simulink model "hp_v5"  (R2024a)
settings: Solver=VariableStepAuto  StartTime=0.0  StopTime=tf  MaxStep=1e-4  RelTol=1e-3  AbsTol=1e-4
values from neighbouring files (symbols this model uses):
  coupler = hexapod.coupler    [calcMotorAngles.m]    (also in calcMotorAngles2.m; calcMotorAngles3.m; calcQ.m; calcQ2_bak.m)
  D = 2 * zeta * w_n * J_e    [controller_parameters.m]    (also in main.m; main_feedforward.m)
  excenter = hexapod.excenter    [calcMotorAngles.m]    (also in calcMotorAngles2.m; calcMotorAngles3.m; calcQ.m; calcQ2_bak.m)
  linear_spring_length = 1    [main.m]    (also in main_feedforward.m = 10)
  linear_spring_offset = ((((platform_mass + 6 * coupler_mass+ 6 * excenter_mass/2) * g)) / linear_spring_constant)    [main.m]    (also in main_feedforward.m = ((platform_mass + 6*coupler_mass+ 6 * excenter_mass/2) * g) )
  motorData = [time0, -motorAngles(:,1), -motorAngles(:,2),                -motorAngles(:,3), -motorAngles(:,4),                -motorAngles(:,5), -motorAngles(:,6)]    [calcSpringParam.m]    (also in calc_spring_param.m; generateMotorDataFromFile.m = [time0, -motorAngles(:,1), -motorAngles(:,2),               ; generateMotorDataFromTrajFile.m = [time0, -motorAngles(:,1), -motorAngles(:,2),               ; generateMotorDataJog.m = [time0, -motorAngles(:,1), -motorAngles(:,2),               )
  N = size(M, 1)    [generateMotorDataFromFile.m]    (also in generateMotorDataFromTrajFile.m; main.m = 36; main_feedforward.m = 36; rw.m = size(data, 1))
  P = w_n^2 * J_e - K_e    [controller_parameters.m]    (also in main.m; main_feedforward.m)
  q = q_rots    [q_test.m]
  radius = 0.01    [main.m]    (also in main_feedforward.m)
  w_f = w_n *10    (= 942.477796077)    [controller_parameters.m]    (also in main.m = 837.758040957; main_feedforward.m = 837.758040957)
  Y = fft(motorAnglesmask(:, col))    [calc_spring_param.m]
undefined symbols (not defined in the file or in its folder): X, y_zero, Z
libraries: nesl_utility x54, sm_lib x48
(part 2 of 2)

== system hp_v5/Lookup tables ==
  1-D Lookup Table : Lookup_n-D  NumberOfTableDimensions=1  BreakpointsForDimension1=motorData(:,1)  Table=motorData(:,2)  InterpMethod=Cubic spline  InternalRulePriority=Speed  RndMeth=Simplest
  1-D Lookup Table1 : Lookup_n-D  NumberOfTableDimensions=1  BreakpointsForDimension1=motorData(:,1)  Table=motorData(:,3)  InterpMethod=Cubic spline  InternalRulePriority=Speed  RndMeth=Simplest
  1-D Lookup Table2 : Lookup_n-D  NumberOfTableDimensions=1  BreakpointsForDimension1=motorData(:,1)  Table=motorData(:,4)  InterpMethod=Cubic spline  InternalRulePriority=Speed  RndMeth=Simplest
  1-D Lookup Table3 : Lookup_n-D  NumberOfTableDimensions=1  BreakpointsForDimension1=motorData(:,1)  Table=motorData(:,5)  InterpMethod=Cubic spline  InternalRulePriority=Speed  RndMeth=Simplest
  1-D Lookup Table4 : Lookup_n-D  NumberOfTableDimensions=1  BreakpointsForDimension1=motorData(:,1)  Table=motorData(:,6)  InterpMethod=Cubic spline  InternalRulePriority=Speed  RndMeth=Simplest
  1-D Lookup Table5 : Lookup_n-D  NumberOfTableDimensions=1  BreakpointsForDimension1=motorData(:,1)  Table=motorData(:,7)  InterpMethod=Cubic spline  InternalRulePriority=Speed  RndMeth=Simplest
  Clock : Clock
  Mux1 : Mux  Inputs=6
  Angles : Outport
  wires:
  Mux1/1 -> Angles/1
  1-D Lookup Table5/1 -> Mux1/6  "lookup"
  1-D Lookup Table3/1 -> Mux1/4  "lookup"
  1-D Lookup Table1/1 -> Mux1/2  "lookup"
  Clock/1 -> 1-D Lookup Table/1, 1-D Lookup Table1/1, 1-D Lookup Table2/1, 1-D Lookup Table5/1, 1-D Lookup Table4/1, 1-D Lookup Table3/1
  1-D Lookup Table4/1 -> Mux1/5  "lookup"
  1-D Lookup Table2/1 -> Mux1/3  "lookup"
  1-D Lookup Table/1 -> Mux1/1  "lookup"

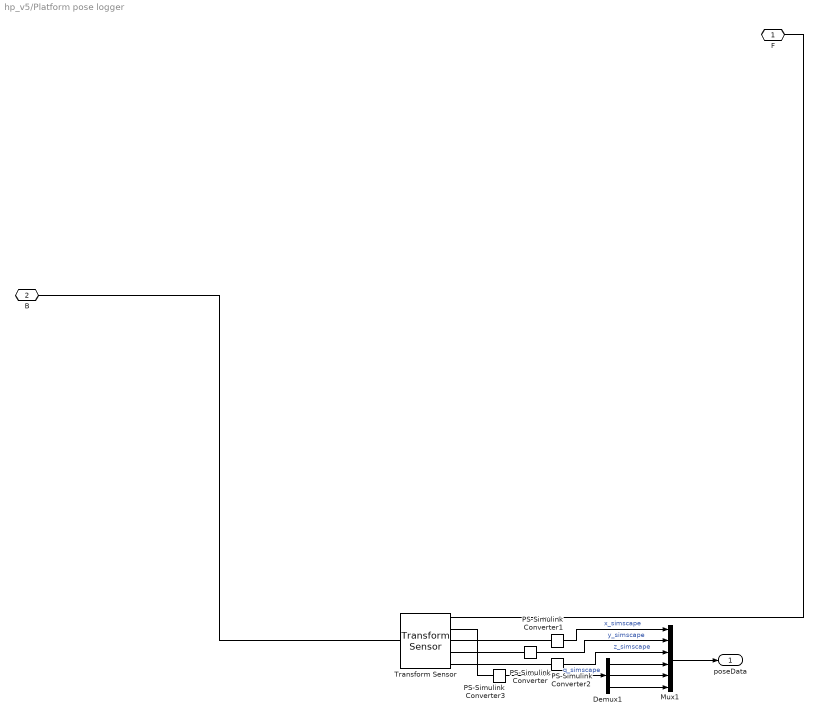
== system hp_v5/Platform pose logger ==
  Demux1 : Demux  Outputs=3
  Mux1 : Mux  Inputs=6
  PS-Simulink Converter{,1..3} (4 alike) : nesl_utility/PS-Simulink Converter  PhysicalDomain=network_engine_domain  SubClassName=ps_output  LeftPortType=input  RightPortType=output  PseudoPeriodic=off  Frequencies=[]  VectorFormat=inherit  Unit=inherit  AffineConversion=off
  Transform Sensor : sm_lib/Frames and Transforms/Transform Sensor  MeasurementFrame=World  RotationSequence=XYZ  SenseAngle=off  SenseAxis=off  SenseQ=off  SenseR=off  SenseRotationSequence=on  SenseOmegaX=off  SenseOmegaY=off  SenseOmegaZ=off  SenseOmega=off  SenseQDot=off  SenseRDot=off  SenseRotationSequenceDot=off  SenseAlphaX=off  SenseAlphaY=off  SenseAlphaZ=off  SenseAlpha=off  SenseQDDot=off  SenseRDDot=off  SenseX=on  SenseY=on  SenseZ=on  SenseXYZ=off  SenseRad=off  SenseAzim=off  SenseDist=off  SenseInc=off  SenseXDot=off  SenseYDot=off  SenseZDot=off  SenseXYZDot=off  SenseRadDot=off  SenseAzimDot=off  SenseDistDot=off  SenseIncDot=off  SenseXDDot=off  SenseYDDot=off  SenseZDDot=off  SenseXYZDDot=off  SenseRadDDot=off  SenseAzimDDot=off  SenseDistDDot=off  SenseIncDDot=off
  F : PMIOPort  Side=Right
  B : PMIOPort  Port=2  Side=Left
  poseData : Outport
  wires:
  Demux1/1 -> Mux1/4
  Demux1/2 -> Mux1/5
  Demux1/3 -> Mux1/6
  PS-Simulink Converter/1 -> Mux1/2  "y_simscape"
  PS-Simulink Converter2/1 -> Mux1/3  "z_simscape"
  PS-Simulink Converter1/1 -> Mux1/1  "x_simscape"
  PS-Simulink Converter3/1 -> Demux1/1  "q_simscape"
  Mux1/1 -> poseData/1
  connections:
  PS-Simulink Converter2/LConn1 -- Transform Sensor/RConn5
  PS-Simulink Converter/LConn1 -- Transform Sensor/RConn4
  PS-Simulink Converter1/LConn1 -- Transform Sensor/RConn3
  PS-Simulink Converter3/LConn1 -- Transform Sensor/RConn2
  Transform Sensor/LConn1 -- B/RConn1
  F/RConn1 -- Transform Sensor/RConn1

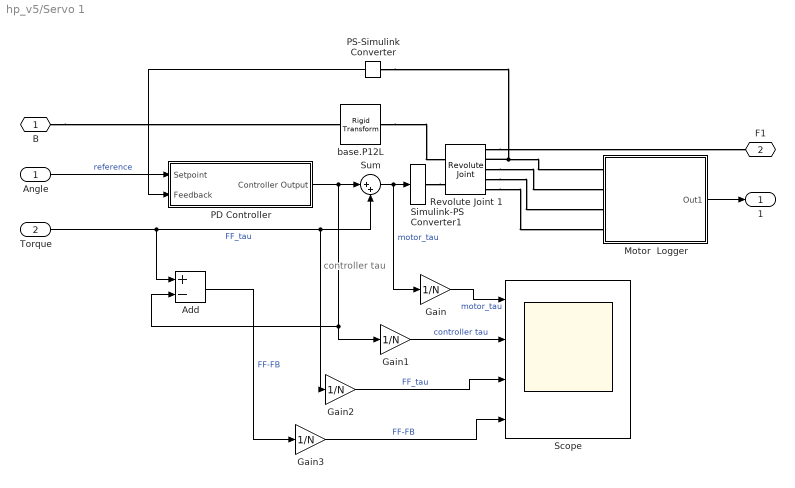
== system hp_v5/Servo 1 ==
  note: controller tau
  Angle : Inport
  Torque : Inport  Port=2
  Add : Sum  Inputs=+-
  Gain{,1..3} (4 alike) : Gain  Gain=1/N
  Motor  Logger : Subsystem
  PD Controller : Subsystem
  PS-Simulink Converter : nesl_utility/PS-Simulink Converter  PhysicalDomain=network_engine_domain  SubClassName=ps_output  LeftPortType=input  RightPortType=output  PseudoPeriodic=off  Frequencies=[]  VectorFormat=inherit  Unit=inherit  AffineConversion=off
  Revolute Joint 1 : sm_lib/Joints/Revolute Joint  JointMode=Normal  CompositeWrenchDir=FollowerOnBase  CompositeWrenchFrame=BaseFrame  SenseConstraintForce=off  SenseConstraintTorque=off  SenseTotalForce=off  SenseTotalTorque=off  PositionTargetSpecify=off  PositionTargetPriority=High  PositionTargetValue=0  PositionTargetValueUnits=deg  VelocityTargetSpecify=off  VelocityTargetPriority=High  VelocityTargetValue=0  VelocityTargetValueUnits=deg/s  EquilibriumPosition=0  EquilibriumPositionUnits=rad  SpringStiffness=0  SpringStiffnessUnits=N*m/rad  DampingCoefficient=0  DampingCoefficientUnits=N*m*s/rad  LowerLimitSpecify=off  LowerLimitBound=-90  LowerLimitBoundUnits=deg  LowerLimitStiffness=1e4  LowerLimitStiffnessUnits=N*m/deg  LowerLimitDamping=10  LowerLimitDampingUnits=N*m/(deg/s)  LowerLimitTransitionRegionWidth=0.1  LowerLimitTransitionRegionWidthUnits=deg  UpperLimitSpecify=off  UpperLimitBound=90  UpperLimitBoundUnits=deg  UpperLimitStiffness=1e4  UpperLimitStiffnessUnits=N*m/deg  UpperLimitDamping=10  UpperLimitDampingUnits=N*m/(deg/s)  UpperLimitTransitionRegionWidth=0.1  UpperLimitTransitionRegionWidthUnits=deg  TorqueActuationMode=InputTorque  MotionActuationMode=ComputedMotion  SensePosition=on  SenseVelocity=on  SenseAcceleration=on  SenseTorqueForce=on  SenseLowerLimitTorqueForce=off  SenseUpperLimitTorqueForce=off
  Scope : Scope  NumInputPorts=4
  Simulink-PS Converter1 : nesl_utility/Simulink-PS Converter  PhysicalDomain=network_engine_domain  SubClassName=ps_input  LeftPortType=input  RightPortType=output  PseudoPeriodic=off  Frequencies=[]  NoiseDistribution=none  NoiseParameters=[]  Unit=1  AffineConversion=off  FilteringAndDerivatives=filter  SimscapeFilterOrder=2  InputFilterTimeConstant=0.001  UdotUserProvided=1
  Sum : Sum  Inputs=|++
  base.P12L : sm_lib/Frames and Transforms/Rigid Transform  RotationMethod=StandardAxis  FollAlignAxisA=+X  BaseAlignAxisA=+Y  FollAlignAxisB=+Y  BaseAlignAxisB=+Z  RotationStandardAxis=+Y  RotationAngle=-120  RotationAngleUnits=deg  RotationArbitraryAxis=[0 0 1]  RotationSequenceAxes=FollowerAxes  RotationSequence=XYX  RotationSequenceAngles=[0 0 0]  RotationSequenceAnglesUnits=deg  RotationMatrix=[1 0 0;0 1 0;0 0 1]  Quaternion=[1 0 0 0]  TranslationMethod=Cartesian  TranslationCartesianOffset=base.P12L  TranslationCartesianOffsetUnits=m  TranslationStandardAxis=+Z  TranslationStandardOffset=0  TranslationStandardOffsetUnits=m  TranslationROffset=0  TranslationROffsetUnits=m  TranslationThetaOffset=0  TranslationThetaOffsetUnits=deg  TranslationZOffset=0  TranslationZOffsetUnits=m
  B : PMIOPort  Side=Left
  F1 : PMIOPort  Port=2  Side=Right
  1 : Outport
  wires:
  PS-Simulink Converter/1 -> PD Controller/2(Feedback)
  Angle/1 -> PD Controller/1(Setpoint)  "reference"
  PD Controller/1(Controller Output) -> Add/2, Gain1/1, Sum/1
  Motor  Logger/1(Out1) -> 1/1
  Torque/1 -> Add/1, Gain2/1, Sum/2  "FF_tau"
  Sum/1 -> Gain/1, Simulink-PS Converter1/1  "motor_tau"
  Add/1 -> Gain3/1  "FF-FB"
  Gain/1 -> Scope/1  "motor_tau"
  Gain1/1 -> Scope/2  "controller tau"
  Gain2/1 -> Scope/3  "FF_tau"
  Gain3/1 -> Scope/4  "FF-FB"
  connections:
  Revolute Joint 1/RConn1 -- F1/RConn1
  Revolute Joint 1/RConn5 -- Motor  Logger/LConn4
  PS-Simulink Converter/LConn1 -- Motor  Logger/LConn1 -- Revolute Joint 1/RConn2
  Simulink-PS Converter1/RConn1 -- Revolute Joint 1/LConn2
  base.P12L/RConn1 -- Revolute Joint 1/LConn1
  B/RConn1 -- base.P12L/LConn1
  Revolute Joint 1/RConn3 -- Motor  Logger/LConn2
  Revolute Joint 1/RConn4 -- Motor  Logger/LConn3

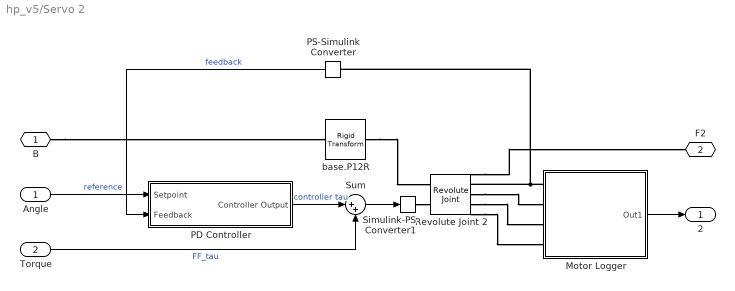
== system hp_v5/Servo 2 ==
  Angle : Inport
  Torque : Inport  Port=2
  Motor Logger : Subsystem
  PD Controller : Subsystem
  PS-Simulink Converter : nesl_utility/PS-Simulink Converter  PhysicalDomain=network_engine_domain  SubClassName=ps_output  LeftPortType=input  RightPortType=output  PseudoPeriodic=off  Frequencies=[]  VectorFormat=inherit  Unit=inherit  AffineConversion=off
  Revolute Joint 2 : sm_lib/Joints/Revolute Joint  JointMode=Normal  CompositeWrenchDir=FollowerOnBase  CompositeWrenchFrame=BaseFrame  SenseConstraintForce=off  SenseConstraintTorque=off  SenseTotalForce=off  SenseTotalTorque=off  PositionTargetSpecify=off  PositionTargetPriority=High  PositionTargetValue=0  PositionTargetValueUnits=deg  VelocityTargetSpecify=off  VelocityTargetPriority=High  VelocityTargetValue=0  VelocityTargetValueUnits=deg/s  EquilibriumPosition=0  EquilibriumPositionUnits=rad  SpringStiffness=0  SpringStiffnessUnits=N*m/rad  DampingCoefficient=0  DampingCoefficientUnits=N*m/(deg/s)  LowerLimitSpecify=off  LowerLimitBound=-90  LowerLimitBoundUnits=deg  LowerLimitStiffness=1e4  LowerLimitStiffnessUnits=N*m/deg  LowerLimitDamping=10  LowerLimitDampingUnits=N*m/(deg/s)  LowerLimitTransitionRegionWidth=0.1  LowerLimitTransitionRegionWidthUnits=deg  UpperLimitSpecify=off  UpperLimitBound=90  UpperLimitBoundUnits=deg  UpperLimitStiffness=1e4  UpperLimitStiffnessUnits=N*m/deg  UpperLimitDamping=10  UpperLimitDampingUnits=N*m/(deg/s)  UpperLimitTransitionRegionWidth=0.1  UpperLimitTransitionRegionWidthUnits=deg  TorqueActuationMode=InputTorque  MotionActuationMode=ComputedMotion  SensePosition=on  SenseVelocity=on  SenseAcceleration=on  SenseTorqueForce=on  SenseLowerLimitTorqueForce=off  SenseUpperLimitTorqueForce=off
  Simulink-PS Converter1 : nesl_utility/Simulink-PS Converter  PhysicalDomain=network_engine_domain  SubClassName=ps_input  LeftPortType=input  RightPortType=output  PseudoPeriodic=off  Frequencies=[]  NoiseDistribution=none  NoiseParameters=[]  Unit=1  AffineConversion=off  FilteringAndDerivatives=filter  SimscapeFilterOrder=2  InputFilterTimeConstant=0.001  UdotUserProvided=0
  Sum : Sum  Inputs=|++
  base.P12R : sm_lib/Frames and Transforms/Rigid Transform  RotationMethod=StandardAxis  FollAlignAxisA=+X  BaseAlignAxisA=+Y  FollAlignAxisB=+Y  BaseAlignAxisB=+Z  RotationStandardAxis=+Y  RotationAngle=60  RotationAngleUnits=deg  RotationArbitraryAxis=[0 0 1]  RotationSequenceAxes=FollowerAxes  RotationSequence=XYX  RotationSequenceAngles=[0 0 0]  RotationSequenceAnglesUnits=deg  RotationMatrix=[1 0 0;0 1 0;0 0 1]  Quaternion=[1 0 0 0]  TranslationMethod=Cartesian  TranslationCartesianOffset=base.P12R  TranslationCartesianOffsetUnits=m  TranslationStandardAxis=+Z  TranslationStandardOffset=0  TranslationStandardOffsetUnits=m  TranslationROffset=0  TranslationROffsetUnits=m  TranslationThetaOffset=0  TranslationThetaOffsetUnits=deg  TranslationZOffset=0  TranslationZOffsetUnits=m
  B : PMIOPort  Side=Left
  F2 : PMIOPort  Port=2  Side=Right
  2 : Outport
  wires:
  Angle/1 -> PD Controller/1(Setpoint)  "reference"
  PD Controller/1(Controller Output) -> Sum/1  "controller tau"
  PS-Simulink Converter/1 -> PD Controller/2(Feedback)  "feedback"
  Motor Logger/1(Out1) -> 2/1
  Sum/1 -> Simulink-PS Converter1/1
  Torque/1 -> Sum/2  "FF_tau"
  connections:
  Revolute Joint 2/RConn1 -- F2/RConn1
  base.P12R/RConn1 -- Revolute Joint 2/LConn1
  Revolute Joint 2/RConn5 -- Motor Logger/LConn4
  Simulink-PS Converter1/RConn1 -- Revolute Joint 2/LConn2
  B/RConn1 -- base.P12R/LConn1
  Revolute Joint 2/RConn3 -- Motor Logger/LConn2
  Revolute Joint 2/RConn4 -- Motor Logger/LConn3
  Motor Logger/LConn1 -- PS-Simulink Converter/LConn1 -- Revolute Joint 2/RConn2

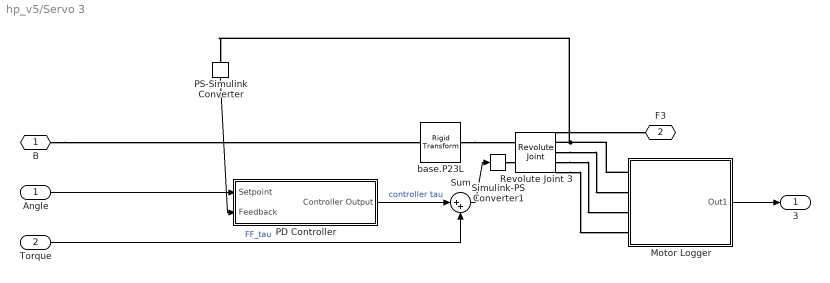
== system hp_v5/Servo 3 ==
  Angle : Inport
  Torque : Inport  Port=2
  Motor Logger : Subsystem
  PD Controller : Subsystem
  PS-Simulink Converter : nesl_utility/PS-Simulink Converter  PhysicalDomain=network_engine_domain  SubClassName=ps_output  LeftPortType=input  RightPortType=output  PseudoPeriodic=off  Frequencies=[]  VectorFormat=inherit  Unit=inherit  AffineConversion=off
  Revolute Joint 3 : sm_lib/Joints/Revolute Joint  JointMode=Normal  CompositeWrenchDir=FollowerOnBase  CompositeWrenchFrame=BaseFrame  SenseConstraintForce=off  SenseConstraintTorque=off  SenseTotalForce=off  SenseTotalTorque=off  PositionTargetSpecify=off  PositionTargetPriority=High  PositionTargetValue=0  PositionTargetValueUnits=deg  VelocityTargetSpecify=off  VelocityTargetPriority=High  VelocityTargetValue=0  VelocityTargetValueUnits=deg/s  EquilibriumPosition=0  EquilibriumPositionUnits=rad  SpringStiffness=0  SpringStiffnessUnits=N*m/rad  DampingCoefficient=0  DampingCoefficientUnits=N*m/(deg/s)  LowerLimitSpecify=off  LowerLimitBound=-90  LowerLimitBoundUnits=deg  LowerLimitStiffness=1e4  LowerLimitStiffnessUnits=N*m/deg  LowerLimitDamping=10  LowerLimitDampingUnits=N*m/(deg/s)  LowerLimitTransitionRegionWidth=0.1  LowerLimitTransitionRegionWidthUnits=deg  UpperLimitSpecify=off  UpperLimitBound=90  UpperLimitBoundUnits=deg  UpperLimitStiffness=1e4  UpperLimitStiffnessUnits=N*m/deg  UpperLimitDamping=10  UpperLimitDampingUnits=N*m/(deg/s)  UpperLimitTransitionRegionWidth=0.1  UpperLimitTransitionRegionWidthUnits=deg  TorqueActuationMode=InputTorque  MotionActuationMode=ComputedMotion  SensePosition=on  SenseVelocity=on  SenseAcceleration=on  SenseTorqueForce=on  SenseLowerLimitTorqueForce=off  SenseUpperLimitTorqueForce=off
  Simulink-PS Converter1 : nesl_utility/Simulink-PS Converter  PhysicalDomain=network_engine_domain  SubClassName=ps_input  LeftPortType=input  RightPortType=output  PseudoPeriodic=off  Frequencies=[]  NoiseDistribution=none  NoiseParameters=[]  Unit=1  AffineConversion=off  FilteringAndDerivatives=filter  SimscapeFilterOrder=2  InputFilterTimeConstant=0.001  UdotUserProvided=0
  Sum : Sum  Inputs=|++
  base.P23L : sm_lib/Frames and Transforms/Rigid Transform  RotationMethod=StandardAxis  FollAlignAxisA=+X  BaseAlignAxisA=+Y  FollAlignAxisB=+Y  BaseAlignAxisB=+Z  RotationStandardAxis=+Y  RotationAngle=0  RotationAngleUnits=deg  RotationArbitraryAxis=[0 0 1]  RotationSequenceAxes=FollowerAxes  RotationSequence=XYX  RotationSequenceAngles=[0 0 0]  RotationSequenceAnglesUnits=deg  RotationMatrix=[1 0 0;0 1 0;0 0 1]  Quaternion=[1 0 0 0]  TranslationMethod=Cartesian  TranslationCartesianOffset=base.P23L  TranslationCartesianOffsetUnits=m  TranslationStandardAxis=+Z  TranslationStandardOffset=0  TranslationStandardOffsetUnits=m  TranslationROffset=0  TranslationROffsetUnits=m  TranslationThetaOffset=0  TranslationThetaOffsetUnits=deg  TranslationZOffset=0  TranslationZOffsetUnits=m
  B : PMIOPort  Side=Left
  F3 : PMIOPort  Port=2  Side=Right
  3 : Outport
  wires:
  Motor Logger/1(Out1) -> 3/1
  Angle/1 -> PD Controller/1(Setpoint)
  PS-Simulink Converter/1 -> PD Controller/2(Feedback)
  PD Controller/1(Controller Output) -> Sum/1  "controller tau"
  Sum/1 -> Simulink-PS Converter1/1
  Torque/1 -> Sum/2  "FF_tau"
  connections:
  Revolute Joint 3/RConn5 -- Motor Logger/LConn4
  Revolute Joint 3/RConn4 -- Motor Logger/LConn3
  Simulink-PS Converter1/RConn1 -- Revolute Joint 3/LConn2
  Revolute Joint 3/RConn3 -- Motor Logger/LConn2
  B/RConn1 -- base.P23L/LConn1
  Revolute Joint 3/RConn1 -- F3/RConn1
  base.P23L/RConn1 -- Revolute Joint 3/LConn1
  Motor Logger/LConn1 -- PS-Simulink Converter/LConn1 -- Revolute Joint 3/RConn2

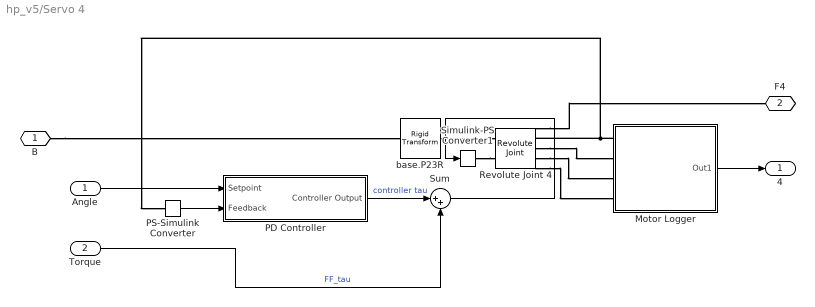
== system hp_v5/Servo 4 ==
  Angle : Inport
  Torque : Inport  Port=2
  Motor Logger : Subsystem
  PD Controller : Subsystem
  PS-Simulink Converter : nesl_utility/PS-Simulink Converter  PhysicalDomain=network_engine_domain  SubClassName=ps_output  LeftPortType=input  RightPortType=output  PseudoPeriodic=off  Frequencies=[]  VectorFormat=inherit  Unit=inherit  AffineConversion=off
  Revolute Joint 4 : sm_lib/Joints/Revolute Joint  JointMode=Normal  CompositeWrenchDir=FollowerOnBase  CompositeWrenchFrame=BaseFrame  SenseConstraintForce=off  SenseConstraintTorque=off  SenseTotalForce=off  SenseTotalTorque=off  PositionTargetSpecify=off  PositionTargetPriority=High  PositionTargetValue=0  PositionTargetValueUnits=deg  VelocityTargetSpecify=off  VelocityTargetPriority=High  VelocityTargetValue=0  VelocityTargetValueUnits=deg/s  EquilibriumPosition=0  EquilibriumPositionUnits=rad  SpringStiffness=0  SpringStiffnessUnits=N*m/rad  DampingCoefficient=0  DampingCoefficientUnits=N*m/(deg/s)  LowerLimitSpecify=off  LowerLimitBound=-90  LowerLimitBoundUnits=deg  LowerLimitStiffness=1e4  LowerLimitStiffnessUnits=N*m/deg  LowerLimitDamping=10  LowerLimitDampingUnits=N*m/(deg/s)  LowerLimitTransitionRegionWidth=0.1  LowerLimitTransitionRegionWidthUnits=deg  UpperLimitSpecify=off  UpperLimitBound=90  UpperLimitBoundUnits=deg  UpperLimitStiffness=1e4  UpperLimitStiffnessUnits=N*m/deg  UpperLimitDamping=10  UpperLimitDampingUnits=N*m/(deg/s)  UpperLimitTransitionRegionWidth=0.1  UpperLimitTransitionRegionWidthUnits=deg  TorqueActuationMode=InputTorque  MotionActuationMode=ComputedMotion  SensePosition=on  SenseVelocity=on  SenseAcceleration=on  SenseTorqueForce=on  SenseLowerLimitTorqueForce=off  SenseUpperLimitTorqueForce=off
  Simulink-PS Converter1 : nesl_utility/Simulink-PS Converter  PhysicalDomain=network_engine_domain  SubClassName=ps_input  LeftPortType=input  RightPortType=output  PseudoPeriodic=off  Frequencies=[]  NoiseDistribution=none  NoiseParameters=[]  Unit=1  AffineConversion=off  FilteringAndDerivatives=filter  SimscapeFilterOrder=2  InputFilterTimeConstant=0.001  UdotUserProvided=0
  Sum : Sum  Inputs=|++
  base.P23R : sm_lib/Frames and Transforms/Rigid Transform  RotationMethod=StandardAxis  FollAlignAxisA=+X  BaseAlignAxisA=+Y  FollAlignAxisB=+Y  BaseAlignAxisB=+Z  RotationStandardAxis=+Y  RotationAngle=180  RotationAngleUnits=deg  RotationArbitraryAxis=[0 0 1]  RotationSequenceAxes=FollowerAxes  RotationSequence=XYX  RotationSequenceAngles=[0 0 0]  RotationSequenceAnglesUnits=deg  RotationMatrix=[1 0 0;0 1 0;0 0 1]  Quaternion=[1 0 0 0]  TranslationMethod=Cartesian  TranslationCartesianOffset=base.P23R  TranslationCartesianOffsetUnits=m  TranslationStandardAxis=+Z  TranslationStandardOffset=0  TranslationStandardOffsetUnits=m  TranslationROffset=0  TranslationROffsetUnits=m  TranslationThetaOffset=0  TranslationThetaOffsetUnits=deg  TranslationZOffset=0  TranslationZOffsetUnits=m
  B : PMIOPort  Side=Left
  F4 : PMIOPort  Port=2  Side=Right
  4 : Outport
  wires:
  PD Controller/1(Controller Output) -> Sum/1  "controller tau"
  Motor Logger/1(Out1) -> 4/1
  Angle/1 -> PD Controller/1(Setpoint)
  PS-Simulink Converter/1 -> PD Controller/2(Feedback)
  Torque/1 -> Sum/2  "FF_tau"
  Sum/1 -> Simulink-PS Converter1/1
  connections:
  Revolute Joint 4/RConn4 -- Motor Logger/LConn3
  B/RConn1 -- base.P23R/LConn1
  base.P23R/RConn1 -- Revolute Joint 4/LConn1
  Revolute Joint 4/RConn3 -- Motor Logger/LConn2
  Simulink-PS Converter1/RConn1 -- Revolute Joint 4/LConn2
  Revolute Joint 4/RConn5 -- Motor Logger/LConn4
  Revolute Joint 4/RConn1 -- F4/RConn1
  Motor Logger/LConn1 -- PS-Simulink Converter/LConn1 -- Revolute Joint 4/RConn2

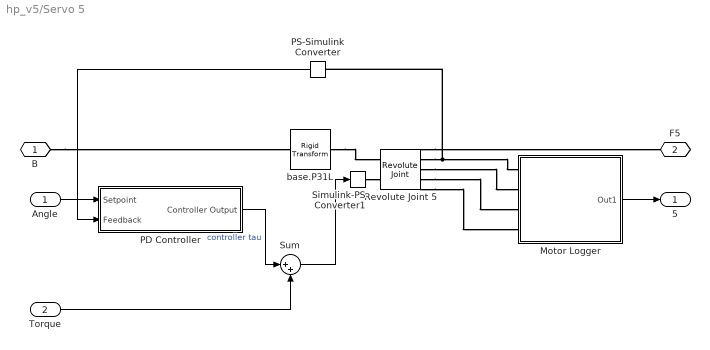
== system hp_v5/Servo 5 ==
  Angle : Inport
  Torque : Inport  Port=2
  Motor Logger : Subsystem
  PD Controller : Subsystem
  PS-Simulink Converter : nesl_utility/PS-Simulink Converter  PhysicalDomain=network_engine_domain  SubClassName=ps_output  LeftPortType=input  RightPortType=output  PseudoPeriodic=off  Frequencies=[]  VectorFormat=inherit  Unit=inherit  AffineConversion=off
  Revolute Joint 5 : sm_lib/Joints/Revolute Joint  JointMode=Normal  CompositeWrenchDir=FollowerOnBase  CompositeWrenchFrame=BaseFrame  SenseConstraintForce=off  SenseConstraintTorque=off  SenseTotalForce=off  SenseTotalTorque=off  PositionTargetSpecify=off  PositionTargetPriority=High  PositionTargetValue=0  PositionTargetValueUnits=deg  VelocityTargetSpecify=off  VelocityTargetPriority=High  VelocityTargetValue=0  VelocityTargetValueUnits=deg/s  EquilibriumPosition=0  EquilibriumPositionUnits=rad  SpringStiffness=0  SpringStiffnessUnits=N*m/rad  DampingCoefficient=0  DampingCoefficientUnits=N*m/(deg/s)  LowerLimitSpecify=off  LowerLimitBound=-90  LowerLimitBoundUnits=deg  LowerLimitStiffness=1e4  LowerLimitStiffnessUnits=N*m/deg  LowerLimitDamping=10  LowerLimitDampingUnits=N*m/(deg/s)  LowerLimitTransitionRegionWidth=0.1  LowerLimitTransitionRegionWidthUnits=deg  UpperLimitSpecify=off  UpperLimitBound=90  UpperLimitBoundUnits=deg  UpperLimitStiffness=1e4  UpperLimitStiffnessUnits=N*m/deg  UpperLimitDamping=10  UpperLimitDampingUnits=N*m/(deg/s)  UpperLimitTransitionRegionWidth=0.1  UpperLimitTransitionRegionWidthUnits=deg  TorqueActuationMode=InputTorque  MotionActuationMode=ComputedMotion  SensePosition=on  SenseVelocity=on  SenseAcceleration=on  SenseTorqueForce=on  SenseLowerLimitTorqueForce=off  SenseUpperLimitTorqueForce=off
  Simulink-PS Converter1 : nesl_utility/Simulink-PS Converter  PhysicalDomain=network_engine_domain  SubClassName=ps_input  LeftPortType=input  RightPortType=output  PseudoPeriodic=off  Frequencies=[]  NoiseDistribution=none  NoiseParameters=[]  Unit=1  AffineConversion=off  FilteringAndDerivatives=filter  SimscapeFilterOrder=2  InputFilterTimeConstant=0.001  UdotUserProvided=0
  Sum : Sum  Inputs=|++
  base.P31L : sm_lib/Frames and Transforms/Rigid Transform  RotationMethod=StandardAxis  FollAlignAxisA=+X  BaseAlignAxisA=+Y  FollAlignAxisB=+Y  BaseAlignAxisB=+Z  RotationStandardAxis=+Y  RotationAngle=120  RotationAngleUnits=deg  RotationArbitraryAxis=[0 0 1]  RotationSequenceAxes=FollowerAxes  RotationSequence=XYX  RotationSequenceAngles=[0 0 0]  RotationSequenceAnglesUnits=deg  RotationMatrix=[1 0 0;0 1 0;0 0 1]  Quaternion=[1 0 0 0]  TranslationMethod=Cartesian  TranslationCartesianOffset=base.P31L  TranslationCartesianOffsetUnits=m  TranslationStandardAxis=+Z  TranslationStandardOffset=0  TranslationStandardOffsetUnits=m  TranslationROffset=0  TranslationROffsetUnits=m  TranslationThetaOffset=0  TranslationThetaOffsetUnits=deg  TranslationZOffset=0  TranslationZOffsetUnits=m
  B : PMIOPort  Side=Left
  F5 : PMIOPort  Port=2  Side=Right
  5 : Outport
  wires:
  Angle/1 -> PD Controller/1(Setpoint)
  PD Controller/1(Controller Output) -> Sum/1  "controller tau"
  PS-Simulink Converter/1 -> PD Controller/2(Feedback)
  Motor Logger/1(Out1) -> 5/1
  Sum/1 -> Simulink-PS Converter1/1
  Torque/1 -> Sum/2
  connections:
  B/RConn1 -- base.P31L/LConn1
  Revolute Joint 5/RConn2 -- Motor Logger/LConn1 -- PS-Simulink Converter/LConn1
  base.P31L/RConn1 -- Revolute Joint 5/LConn1
  Simulink-PS Converter1/RConn1 -- Revolute Joint 5/LConn2
  Revolute Joint 5/RConn1 -- F5/RConn1
  Revolute Joint 5/RConn3 -- Motor Logger/LConn2
  Revolute Joint 5/RConn4 -- Motor Logger/LConn3
  Revolute Joint 5/RConn5 -- Motor Logger/LConn4

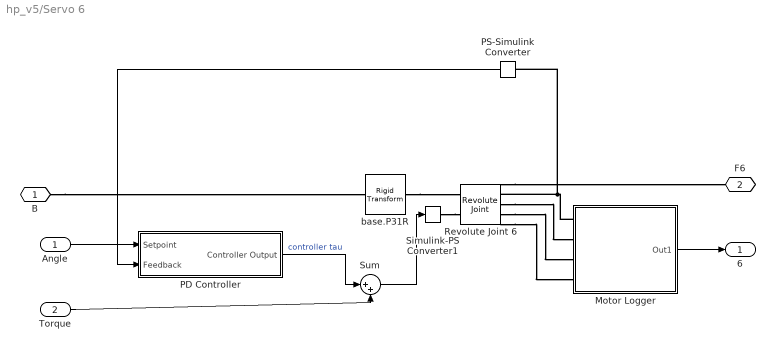
== system hp_v5/Servo 6 ==
  Angle : Inport
  Torque : Inport  Port=2
  Motor Logger : Subsystem
  PD Controller : Subsystem
  PS-Simulink Converter : nesl_utility/PS-Simulink Converter  PhysicalDomain=network_engine_domain  SubClassName=ps_output  LeftPortType=input  RightPortType=output  PseudoPeriodic=off  Frequencies=[]  VectorFormat=inherit  Unit=inherit  AffineConversion=off
  Revolute Joint 6 : sm_lib/Joints/Revolute Joint  JointMode=Normal  CompositeWrenchDir=FollowerOnBase  CompositeWrenchFrame=BaseFrame  SenseConstraintForce=off  SenseConstraintTorque=off  SenseTotalForce=off  SenseTotalTorque=off  PositionTargetSpecify=off  PositionTargetPriority=High  PositionTargetValue=0  PositionTargetValueUnits=deg  VelocityTargetSpecify=off  VelocityTargetPriority=High  VelocityTargetValue=0  VelocityTargetValueUnits=deg/s  EquilibriumPosition=0  EquilibriumPositionUnits=rad  SpringStiffness=0  SpringStiffnessUnits=N*m/rad  DampingCoefficient=0  DampingCoefficientUnits=N*m/(deg/s)  LowerLimitSpecify=off  LowerLimitBound=-90  LowerLimitBoundUnits=deg  LowerLimitStiffness=1e4  LowerLimitStiffnessUnits=N*m/deg  LowerLimitDamping=10  LowerLimitDampingUnits=N*m/(deg/s)  LowerLimitTransitionRegionWidth=0.1  LowerLimitTransitionRegionWidthUnits=deg  UpperLimitSpecify=off  UpperLimitBound=90  UpperLimitBoundUnits=deg  UpperLimitStiffness=1e4  UpperLimitStiffnessUnits=N*m/deg  UpperLimitDamping=10  UpperLimitDampingUnits=N*m/(deg/s)  UpperLimitTransitionRegionWidth=0.1  UpperLimitTransitionRegionWidthUnits=deg  TorqueActuationMode=InputTorque  MotionActuationMode=ComputedMotion  SensePosition=on  SenseVelocity=on  SenseAcceleration=on  SenseTorqueForce=on  SenseLowerLimitTorqueForce=off  SenseUpperLimitTorqueForce=off
  Simulink-PS Converter1 : nesl_utility/Simulink-PS Converter  PhysicalDomain=network_engine_domain  SubClassName=ps_input  LeftPortType=input  RightPortType=output  PseudoPeriodic=off  Frequencies=[]  NoiseDistribution=none  NoiseParameters=[]  Unit=1  AffineConversion=off  FilteringAndDerivatives=filter  SimscapeFilterOrder=2  InputFilterTimeConstant=0.001  UdotUserProvided=0
  Sum : Sum  Inputs=|++
  base.P31R : sm_lib/Frames and Transforms/Rigid Transform  RotationMethod=StandardAxis  FollAlignAxisA=+X  BaseAlignAxisA=+Y  FollAlignAxisB=+Y  BaseAlignAxisB=+Z  RotationStandardAxis=+Y  RotationAngle=300  RotationAngleUnits=deg  RotationArbitraryAxis=[0 0 1]  RotationSequenceAxes=FollowerAxes  RotationSequence=XYX  RotationSequenceAngles=[0 0 0]  RotationSequenceAnglesUnits=deg  RotationMatrix=[1 0 0;0 1 0;0 0 1]  Quaternion=[1 0 0 0]  TranslationMethod=Cartesian  TranslationCartesianOffset=base.P31R  TranslationCartesianOffsetUnits=m  TranslationStandardAxis=+Z  TranslationStandardOffset=0  TranslationStandardOffsetUnits=m  TranslationROffset=0  TranslationROffsetUnits=m  TranslationThetaOffset=0  TranslationThetaOffsetUnits=deg  TranslationZOffset=0  TranslationZOffsetUnits=m
  B : PMIOPort  Side=Left
  F6 : PMIOPort  Port=2  Side=Right
  6 : Outport
  wires:
  PD Controller/1(Controller Output) -> Sum/1  "controller tau"
  Motor Logger/1(Out1) -> 6/1
  Angle/1 -> PD Controller/1(Setpoint)
  PS-Simulink Converter/1 -> PD Controller/2(Feedback)
  Torque/1 -> Sum/2
  Sum/1 -> Simulink-PS Converter1/1
  connections:
  Revolute Joint 6/RConn4 -- Motor Logger/LConn3
  B/RConn1 -- base.P31R/LConn1
  Motor Logger/LConn1 -- Revolute Joint 6/RConn2 -- PS-Simulink Converter/LConn1
  Revolute Joint 6/RConn5 -- Motor Logger/LConn4
  Revolute Joint 6/RConn1 -- F6/RConn1
  base.P31R/RConn1 -- Revolute Joint 6/LConn1
  Revolute Joint 6/RConn3 -- Motor Logger/LConn2
  Simulink-PS Converter1/RConn1 -- Revolute Joint 6/LConn2

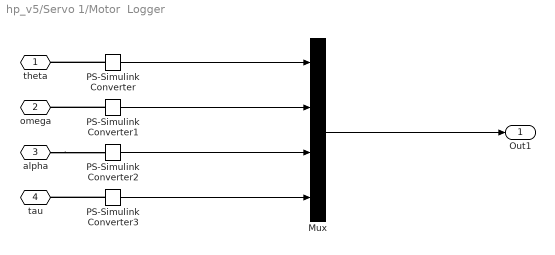
== system hp_v5/Servo 1/Motor  Logger ==
  Mux : Mux
  PS-Simulink Converter{,1..3} (4 alike) : nesl_utility/PS-Simulink Converter  PhysicalDomain=network_engine_domain  SubClassName=ps_output  LeftPortType=input  RightPortType=output  PseudoPeriodic=off  Frequencies=[]  VectorFormat=inherit  Unit=inherit  AffineConversion=off
  theta : PMIOPort  Side=Left
  omega : PMIOPort  Port=2  Side=Left
  alpha : PMIOPort  Port=3  Side=Left
  tau : PMIOPort  Port=4  Side=Left
  Out1 : Outport
  wires:
  PS-Simulink Converter/1 -> Mux/1
  PS-Simulink Converter1/1 -> Mux/2
  PS-Simulink Converter2/1 -> Mux/3
  PS-Simulink Converter3/1 -> Mux/4
  Mux/1 -> Out1/1
  connections:
  PS-Simulink Converter/LConn1 -- theta/RConn1
  PS-Simulink Converter1/LConn1 -- omega/RConn1
  alpha/RConn1 -- PS-Simulink Converter2/LConn1
  PS-Simulink Converter3/LConn1 -- tau/RConn1

== system hp_v5/Servo 1/PD Controller ==
  Setpoint : Inport
  Feedback : Inport  Port=2
  Differentiator : TransferFcn  Numerator=[D*w_f 0]  Denominator=[1 w_f]
  Gain : Gain  Gain=P
  Sum : Sum  Inputs=|+-
  Sum1 : Sum  Inputs=|++
  Controller Output : Outport
  wires:
  Differentiator/1 -> Sum1/2
  Setpoint/1 -> Sum/1
  Gain/1 -> Sum1/1
  Sum1/1 -> Controller Output/1
  Feedback/1 -> Sum/2
  Sum/1 -> Differentiator/1, Gain/1

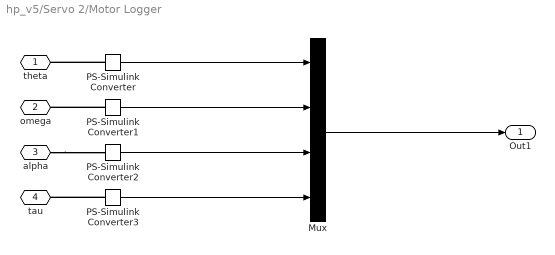
== system hp_v5/Servo 2/Motor Logger ==
  Mux : Mux
  PS-Simulink Converter{,1..3} (4 alike) : nesl_utility/PS-Simulink Converter  PhysicalDomain=network_engine_domain  SubClassName=ps_output  LeftPortType=input  RightPortType=output  PseudoPeriodic=off  Frequencies=[]  VectorFormat=inherit  Unit=inherit  AffineConversion=off
  theta : PMIOPort  Side=Left
  omega : PMIOPort  Port=2  Side=Left
  alpha : PMIOPort  Port=3  Side=Left
  tau : PMIOPort  Port=4  Side=Left
  Out1 : Outport
  wires:
  PS-Simulink Converter/1 -> Mux/1
  PS-Simulink Converter1/1 -> Mux/2
  PS-Simulink Converter2/1 -> Mux/3
  PS-Simulink Converter3/1 -> Mux/4
  Mux/1 -> Out1/1
  connections:
  PS-Simulink Converter/LConn1 -- theta/RConn1
  PS-Simulink Converter1/LConn1 -- omega/RConn1
  alpha/RConn1 -- PS-Simulink Converter2/LConn1
  PS-Simulink Converter3/LConn1 -- tau/RConn1

== system hp_v5/Servo 2/PD Controller ==
  Setpoint : Inport
  Feedback : Inport  Port=2
  Differentiator : TransferFcn  Numerator=[D*w_f 0]  Denominator=[1 w_f]
  Gain : Gain  Gain=P
  Sum : Sum  Inputs=|+-
  Sum1 : Sum  Inputs=|++
  Controller Output : Outport
  wires:
  Differentiator/1 -> Sum1/2
  Setpoint/1 -> Sum/1
  Gain/1 -> Sum1/1
  Sum1/1 -> Controller Output/1
  Feedback/1 -> Sum/2
  Sum/1 -> Differentiator/1, Gain/1

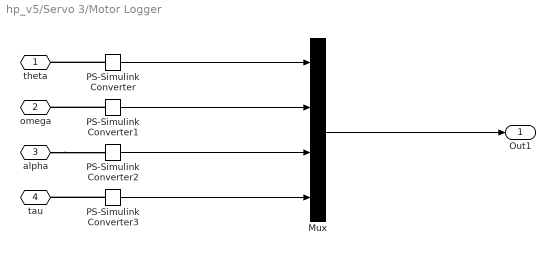
== system hp_v5/Servo 3/Motor Logger ==
  Mux : Mux
  PS-Simulink Converter{,1..3} (4 alike) : nesl_utility/PS-Simulink Converter  PhysicalDomain=network_engine_domain  SubClassName=ps_output  LeftPortType=input  RightPortType=output  PseudoPeriodic=off  Frequencies=[]  VectorFormat=inherit  Unit=inherit  AffineConversion=off
  theta : PMIOPort  Side=Left
  omega : PMIOPort  Port=2  Side=Left
  alpha : PMIOPort  Port=3  Side=Left
  tau : PMIOPort  Port=4  Side=Left
  Out1 : Outport
  wires:
  PS-Simulink Converter/1 -> Mux/1
  PS-Simulink Converter1/1 -> Mux/2
  PS-Simulink Converter2/1 -> Mux/3
  PS-Simulink Converter3/1 -> Mux/4
  Mux/1 -> Out1/1
  connections:
  PS-Simulink Converter/LConn1 -- theta/RConn1
  PS-Simulink Converter1/LConn1 -- omega/RConn1
  alpha/RConn1 -- PS-Simulink Converter2/LConn1
  PS-Simulink Converter3/LConn1 -- tau/RConn1

== system hp_v5/Servo 3/PD Controller ==
  Setpoint : Inport
  Feedback : Inport  Port=2
  Differentiator : TransferFcn  Numerator=[D*w_f 0]  Denominator=[1 w_f]
  Gain : Gain  Gain=P
  Sum : Sum  Inputs=|+-
  Sum1 : Sum  Inputs=|++
  Controller Output : Outport
  wires:
  Differentiator/1 -> Sum1/2
  Setpoint/1 -> Sum/1
  Gain/1 -> Sum1/1
  Sum1/1 -> Controller Output/1
  Feedback/1 -> Sum/2
  Sum/1 -> Differentiator/1, Gain/1

== system hp_v5/Servo 4/Motor Logger ==
  Mux : Mux
  PS-Simulink Converter{,1..3} (4 alike) : nesl_utility/PS-Simulink Converter  PhysicalDomain=network_engine_domain  SubClassName=ps_output  LeftPortType=input  RightPortType=output  PseudoPeriodic=off  Frequencies=[]  VectorFormat=inherit  Unit=inherit  AffineConversion=off
  theta : PMIOPort  Side=Left
  omega : PMIOPort  Port=2  Side=Left
  alpha : PMIOPort  Port=3  Side=Left
  tau : PMIOPort  Port=4  Side=Left
  Out1 : Outport
  wires:
  PS-Simulink Converter/1 -> Mux/1
  PS-Simulink Converter1/1 -> Mux/2
  PS-Simulink Converter2/1 -> Mux/3
  PS-Simulink Converter3/1 -> Mux/4
  Mux/1 -> Out1/1
  connections:
  PS-Simulink Converter/LConn1 -- theta/RConn1
  PS-Simulink Converter1/LConn1 -- omega/RConn1
  alpha/RConn1 -- PS-Simulink Converter2/LConn1
  PS-Simulink Converter3/LConn1 -- tau/RConn1

== system hp_v5/Servo 4/PD Controller ==
  Setpoint : Inport
  Feedback : Inport  Port=2
  Differentiator : TransferFcn  Numerator=[D*w_f 0]  Denominator=[1 w_f]
  Gain : Gain  Gain=P
  Sum : Sum  Inputs=|+-
  Sum1 : Sum  Inputs=|++
  Controller Output : Outport
  wires:
  Differentiator/1 -> Sum1/2
  Setpoint/1 -> Sum/1
  Gain/1 -> Sum1/1
  Sum1/1 -> Controller Output/1
  Feedback/1 -> Sum/2
  Sum/1 -> Differentiator/1, Gain/1

== system hp_v5/Servo 5/Motor Logger ==
  Mux : Mux
  PS-Simulink Converter{,1..3} (4 alike) : nesl_utility/PS-Simulink Converter  PhysicalDomain=network_engine_domain  SubClassName=ps_output  LeftPortType=input  RightPortType=output  PseudoPeriodic=off  Frequencies=[]  VectorFormat=inherit  Unit=inherit  AffineConversion=off
  theta : PMIOPort  Side=Left
  omega : PMIOPort  Port=2  Side=Left
  alpha : PMIOPort  Port=3  Side=Left
  tau : PMIOPort  Port=4  Side=Left
  Out1 : Outport
  wires:
  PS-Simulink Converter/1 -> Mux/1
  PS-Simulink Converter1/1 -> Mux/2
  PS-Simulink Converter2/1 -> Mux/3
  PS-Simulink Converter3/1 -> Mux/4
  Mux/1 -> Out1/1
  connections:
  PS-Simulink Converter/LConn1 -- theta/RConn1
  PS-Simulink Converter1/LConn1 -- omega/RConn1
  alpha/RConn1 -- PS-Simulink Converter2/LConn1
  PS-Simulink Converter3/LConn1 -- tau/RConn1

== system hp_v5/Servo 5/PD Controller ==
  Setpoint : Inport
  Feedback : Inport  Port=2
  Differentiator : TransferFcn  Numerator=[D*w_f 0]  Denominator=[1 w_f]
  Gain : Gain  Gain=P
  Sum : Sum  Inputs=|+-
  Sum1 : Sum  Inputs=|++
  Controller Output : Outport
  wires:
  Differentiator/1 -> Sum1/2
  Setpoint/1 -> Sum/1
  Gain/1 -> Sum1/1
  Sum1/1 -> Controller Output/1
  Feedback/1 -> Sum/2
  Sum/1 -> Differentiator/1, Gain/1

== system hp_v5/Servo 6/Motor Logger ==
  Mux : Mux
  PS-Simulink Converter{,1..3} (4 alike) : nesl_utility/PS-Simulink Converter  PhysicalDomain=network_engine_domain  SubClassName=ps_output  LeftPortType=input  RightPortType=output  PseudoPeriodic=off  Frequencies=[]  VectorFormat=inherit  Unit=inherit  AffineConversion=off
  theta : PMIOPort  Side=Left
  omega : PMIOPort  Port=2  Side=Left
  alpha : PMIOPort  Port=3  Side=Left
  tau : PMIOPort  Port=4  Side=Left
  Out1 : Outport
  wires:
  PS-Simulink Converter/1 -> Mux/1
  PS-Simulink Converter1/1 -> Mux/2
  PS-Simulink Converter2/1 -> Mux/3
  PS-Simulink Converter3/1 -> Mux/4
  Mux/1 -> Out1/1
  connections:
  PS-Simulink Converter/LConn1 -- theta/RConn1
  PS-Simulink Converter1/LConn1 -- omega/RConn1
  alpha/RConn1 -- PS-Simulink Converter2/LConn1
  PS-Simulink Converter3/LConn1 -- tau/RConn1

== system hp_v5/Servo 6/PD Controller ==
  Setpoint : Inport
  Feedback : Inport  Port=2
  Differentiator : TransferFcn  Numerator=[D*w_f 0]  Denominator=[1 w_f]
  Gain : Gain  Gain=P
  Sum : Sum  Inputs=|+-
  Sum1 : Sum  Inputs=|++
  Controller Output : Outport
  wires:
  Differentiator/1 -> Sum1/2
  Setpoint/1 -> Sum/1
  Gain/1 -> Sum1/1
  Sum1/1 -> Controller Output/1
  Feedback/1 -> Sum/2
  Sum/1 -> Differentiator/1, Gain/1

== matlab function hp_v5/MATLAB Function ==
  settings: updateMethod=DISCRETE  sampleTime=ts
  data: u input; tf input
function fcn(u, tf)
% Set the resolution for the progress bar
resolution = 5;  % Update progress bar every 5%

% Calculate the percentage complete
percentage = (u / tf) * 100;

% Check if the percentage is a multiple of the resolution
if mod(percentage, resolution) == 0
    % Calculate the number of dots based on the percentage
    strLength = 30;  % Total length of the progress bar
    nDots = floor(percentage / 100 * strLength);
    dotOut = ['[' repmat('=', 1, nDots) repmat('.', 1, strLength - nDots) ']'];
    percentageOut = sprintf(' : %3d%%', int32(floor(percentage)));

    % Create the output string with ">>" prefix
    strOut = ['>> ' dotOut percentageOut];

    % Print the progress bar
    fprintf('%s\n', strOut);  % Print each progress update on a new line
end

% Handle completion
if percentage >= 100
    fprintf('>> Simulation Complete.\n');
end
end
